simulink model "model_verification"  (R2024a)
settings: Solver=VariableStepAuto  StartTime=0.0  StopTime=91  RelTol=1e-3
settings Model: Creator=ommore5807  LastModifiedBy=WickedSkyn
settings RTWCC: GPUComputeCapability=3.5

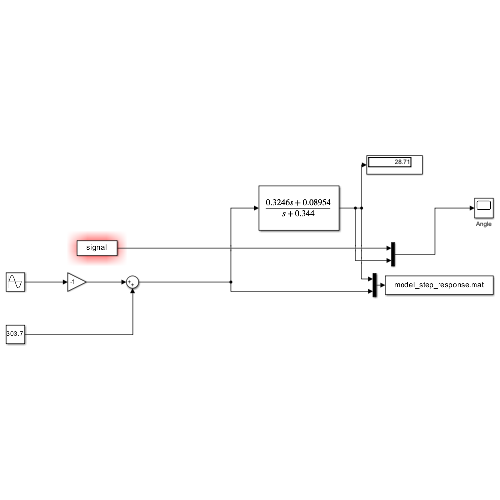
[thumbnail: Simulink's stored preview of the top-level diagram]
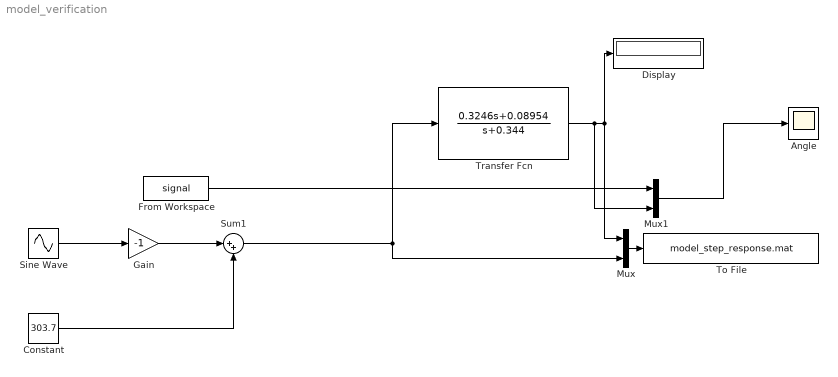
== system model_verification ==
  Angle : Scope
  Constant : Constant  Value=303.7
  Display : Display
  From Workspace : FromWorkspace  VariableName=signal
  Gain : Gain  Gain=-1
  Mux : Mux  Inputs=2
  Mux1 : Mux  Inputs=2
  Sine Wave : Sin  Amplitude=-279.06  Frequency=0.102  Phase=7.105  SampleTime=0
  Sum1 : Sum  Inputs=|++
  To File : ToFile  Filename=model_step_response.mat  MatrixName=model_step_response  SaveFormat=Timeseries
  Transfer Fcn : TransferFcn  Numerator=[0.3246 0.08954]  Denominator=[1 0.344]
  wires:
  Sum1/1 -> Transfer Fcn/1, Mux/2
  Transfer Fcn/1 -> Mux1/2, Display/1, Mux/1
  Mux/1 -> To File/1
  Constant/1 -> Sum1/2
  Mux1/1 -> Angle/1
  From Workspace/1 -> Mux1/1
  Sine Wave/1 -> Gain/1
  Gain/1 -> Sum1/1
